simulink model "IEEE14_case"  (R2024b)
settings: Solver=FixedStepAuto  StartTime=0  StopTime=2  FixedStep=1e-7  RelTol=1e-3
values from neighbouring files (symbols this model uses):
  GFL_15_Bva = 0.009    [IEEE14_parameters.m]
  GFL_15_C_bus_pu = 7.179419    [IEEE14_parameters.m]
  GFL_15_f0 = 60    [IEEE14_parameters.m]
  GFL_15_I_id = 691.26967    [IEEE14_parameters.m]
  GFL_15_I_iq = 691.26967    [IEEE14_parameters.m]
  GFL_15_I_od = 45.2207    [IEEE14_parameters.m]
  GFL_15_I_oq = 45.2207    [IEEE14_parameters.m]
  GFL_15_I_pll = 0.78    [IEEE14_parameters.m]
  GFL_15_Kdi = 0.09    [IEEE14_parameters.m]
  GFL_15_Kdo = 0.9    [IEEE14_parameters.m]
  GFL_15_Kqi = 0.09    [IEEE14_parameters.m]
  GFL_15_Kqo = 0.9    [IEEE14_parameters.m]
  GFL_15_Lg_pu = 0.631447    [IEEE14_parameters.m]
  GFL_15_mode = 1    [IEEE14_parameters.m]
  GFL_15_P_id = 3.7166    [IEEE14_parameters.m]
  GFL_15_P_iq = 3.7166    [IEEE14_parameters.m]
  GFL_15_P_od = 0.4798    [IEEE14_parameters.m]
  GFL_15_P_oq = 0.4798    [IEEE14_parameters.m]
  GFL_15_P_pll = 290.42    [IEEE14_parameters.m]
  GFL_15_Qe_ref = 0.2    [IEEE14_parameters.m]
  GFL_15_Rg_pu = 0.024016    [IEEE14_parameters.m]
  GFL_15_Sbase = 1.000000e+4    (= 10000)    [IEEE14_parameters.m]
  GFL_15_Tdi = 0.01    [IEEE14_parameters.m]
  GFL_15_Tdo = 0.2    [IEEE14_parameters.m]
  GFL_15_Tqi = 0.01    [IEEE14_parameters.m]
  GFL_15_Tqo = 0.2    [IEEE14_parameters.m]
  GFL_15_Vbase = 380    [IEEE14_parameters.m]
  GFL_15_Vdc_ref = 1.011475    [IEEE14_parameters.m]
  GFL_15_Vdcbase = 700    [IEEE14_parameters.m]
  GFL_15_vq_ref = 0    [IEEE14_parameters.m]
  GFL_16_Bva = 0.002    [IEEE14_parameters.m]
  GFL_16_C_bus_pu = 7.179419    [IEEE14_parameters.m]
  GFL_16_f0 = 60    [IEEE14_parameters.m]
  GFL_16_I_id = 691.26967    [IEEE14_parameters.m]
  GFL_16_I_iq = 691.26967    [IEEE14_parameters.m]
  GFL_16_I_od = 45.2207    [IEEE14_parameters.m]
  GFL_16_I_oq = 45.2207    [IEEE14_parameters.m]
  GFL_16_I_pll = 0.78    [IEEE14_parameters.m]
  GFL_16_Kdi = 0.05    [IEEE14_parameters.m]
  GFL_16_Kdo = 0.5    [IEEE14_parameters.m]
  GFL_16_Kqi = 0.05    [IEEE14_parameters.m]
  GFL_16_Kqo = 0.5    [IEEE14_parameters.m]
  GFL_16_Lg_pu = 0.631447    [IEEE14_parameters.m]
  GFL_16_mode = 1    [IEEE14_parameters.m]
  GFL_16_P_id = 3.7166    [IEEE14_parameters.m]
  GFL_16_P_iq = 3.7166    [IEEE14_parameters.m]
  GFL_16_P_od = 0.4798    [IEEE14_parameters.m]
  GFL_16_P_oq = 0.4798    [IEEE14_parameters.m]
  GFL_16_P_pll = 290.42    [IEEE14_parameters.m]
  GFL_16_Qe_ref = 0.2    [IEEE14_parameters.m]
  GFL_16_Rg_pu = 0.024016    [IEEE14_parameters.m]
  GFL_16_Sbase = 1.000000e+4    (= 10000)    [IEEE14_parameters.m]
  GFL_16_Tdi = 0.01    [IEEE14_parameters.m]
  GFL_16_Tdo = 0.2    [IEEE14_parameters.m]
  GFL_16_Tqi = 0.01    [IEEE14_parameters.m]
  GFL_16_Tqo = 0.2    [IEEE14_parameters.m]
  GFL_16_Vbase = 380    [IEEE14_parameters.m]
  GFL_16_Vdc_ref = 1.01144    [IEEE14_parameters.m]
  GFL_16_Vdcbase = 700    [IEEE14_parameters.m]
  GFL_16_vq_ref = 0    [IEEE14_parameters.m]
  GFL_17_Bva = 0.002    [IEEE14_parameters.m]
  GFL_17_C_bus_pu = 7.179419    [IEEE14_parameters.m]
  GFL_17_f0 = 60    [IEEE14_parameters.m]
  GFL_17_I_id = 691.26967    [IEEE14_parameters.m]
  GFL_17_I_iq = 691.26967    [IEEE14_parameters.m]
  GFL_17_I_od = 45.2207    [IEEE14_parameters.m]
  GFL_17_I_oq = 45.2207    [IEEE14_parameters.m]
  GFL_17_I_pll = 0.78    [IEEE14_parameters.m]
  GFL_17_Kdi = 0.05    [IEEE14_parameters.m]
  GFL_17_Kdo = 0.5    [IEEE14_parameters.m]
  GFL_17_Kqi = 0.05    [IEEE14_parameters.m]
  GFL_17_Kqo = 0.5    [IEEE14_parameters.m]
  GFL_17_Lg_pu = 0.631447    [IEEE14_parameters.m]
  GFL_17_mode = 1    [IEEE14_parameters.m]
  GFL_17_P_id = 3.7166    [IEEE14_parameters.m]
  GFL_17_P_iq = 3.7166    [IEEE14_parameters.m]
  GFL_17_P_od = 0.4798    [IEEE14_parameters.m]
  GFL_17_P_oq = 0.4798    [IEEE14_parameters.m]
  GFL_17_P_pll = 290.42    [IEEE14_parameters.m]
  GFL_17_Qe_ref = 0.2    [IEEE14_parameters.m]
  GFL_17_Rg_pu = 0.024016    [IEEE14_parameters.m]
  GFL_17_Sbase = 1.000000e+4    (= 10000)    [IEEE14_parameters.m]
  GFL_17_Tdi = 0.01    [IEEE14_parameters.m]
  GFL_17_Tdo = 0.2    [IEEE14_parameters.m]
  GFL_17_Tqi = 0.01    [IEEE14_parameters.m]
  GFL_17_Tqo = 0.2    [IEEE14_parameters.m]
  GFL_17_Vbase = 380    [IEEE14_parameters.m]
  GFL_17_Vdc_ref = 1.011632    [IEEE14_parameters.m]
  GFL_17_Vdcbase = 700    [IEEE14_parameters.m]
  GFL_17_vq_ref = 0    [IEEE14_parameters.m]
  GFL_18_Bva = 0.002    [IEEE14_parameters.m]
  GFL_18_C_bus_pu = 7.179419    [IEEE14_parameters.m]
  GFL_18_f0 = 60    [IEEE14_parameters.m]
  GFL_18_I_id = 691.26967    [IEEE14_parameters.m]
  GFL_18_I_iq = 691.26967    [IEEE14_parameters.m]
  GFL_18_I_od = 45.2207    [IEEE14_parameters.m]
  GFL_18_I_oq = 45.2207    [IEEE14_parameters.m]
  GFL_18_I_pll = 0.78    [IEEE14_parameters.m]
  GFL_18_Kdi = 0.05    [IEEE14_parameters.m]
  GFL_18_Kdo = 0.5    [IEEE14_parameters.m]
  GFL_18_Kqi = 0.05    [IEEE14_parameters.m]
  GFL_18_Kqo = 0.5    [IEEE14_parameters.m]
  GFL_18_Lg_pu = 0.631447    [IEEE14_parameters.m]
  GFL_18_mode = 1    [IEEE14_parameters.m]
  GFL_18_P_id = 3.7166    [IEEE14_parameters.m]
  GFL_18_P_iq = 3.7166    [IEEE14_parameters.m]
  GFL_18_P_od = 0.4798    [IEEE14_parameters.m]
  GFL_18_P_oq = 0.4798    [IEEE14_parameters.m]
  GFL_18_P_pll = 290.42    [IEEE14_parameters.m]
  GFL_18_Qe_ref = 0.2    [IEEE14_parameters.m]
  GFL_18_Rg_pu = 0.024016    [IEEE14_parameters.m]
  GFL_18_Sbase = 1.000000e+4    (= 10000)    [IEEE14_parameters.m]
  GFL_18_Tdi = 0.01    [IEEE14_parameters.m]
  GFL_18_Tdo = 0.2    [IEEE14_parameters.m]
  GFL_18_Tqi = 0.01    [IEEE14_parameters.m]
  GFL_18_Tqo = 0.2    [IEEE14_parameters.m]
  GFL_18_Vbase = 380    [IEEE14_parameters.m]
  GFL_18_Vdc_ref = 1.011572    [IEEE14_parameters.m]
  GFL_18_Vdcbase = 700    [IEEE14_parameters.m]
  GFL_18_vq_ref = 0    [IEEE14_parameters.m]
  ... (+180 more)
(part 19 of 25)

== system IEEE14_case/SG_D_2/i_q_SG_D_2_block ==
  note: i_q_SG_D_2 in case14gfl
      | $-\frac{\sin\left(\theta _{\mathrm{SG},D,2}\right)\,\left(\psi _{q,\mathrm{SG},D,2}+\frac{\psi _{\mathrm{gq},\mathrm{SG},D,2}\,\left(x_{l}-x_{\mathrm{qdd}}\right)}{x_{l}-x_{\mathrm{qd}}}+\frac{\psi _{\mathrm{kq},\mathrm{SG},D,2}\,\left(x_{\mathrm{qd}}-x_{\mathrm{qdd}}\right)}{x_{l}-x_{\mathrm{qd}}}\right)}{x_{\mathrm{qdd}}}-\frac{\cos\left(\theta _{\mathrm{SG},D,2}\right)\,\left(\frac{\psi _{\mathrm{1d},\mathrm{SG},D,2}\,\left(x_{\mathrm{dd}}-x_{\mathrm{ddd}}\right)}{x_{\mathrm{dd}}-x_{l}}-\psi _{d,\mathrm{SG},D,2}+\frac{\psi _{\mathrm{fd},\mathrm{SG},D,2}\,\left(x_{\mathrm{ddd}}-x_{l}\right)}{x_{\mathrm{dd}}-x_{l}}\right)}{x_{\mathrm{ddd}}}$
      | Automatically generated on 2025-10-09 21:31:35 .
  State_psi_gq_SG_D_2_7930d : Inport
  State_psi_kq_SG_D_2_485e8 : Inport  Port=2
  State_psi_q_SG_D_2_38e4d : Inport  Port=3
  State_theta_SG_D_2_4758d : Inport  Port=4
  State_psi_1d_SG_D_2_da86a : Inport  Port=5
  State_psi_d_SG_D_2_afab4 : Inport  Port=6
  State_psi_fd_SG_D_2_93752 : Inport  Port=7
  State_theta_SG_D_2_47d8a : Inport  Port=8
  Add_21d4d : Sum
  Add_4c702 : Sum
  Add_61a1f : Sum
  Add_93cfc : Sum
  Add_a0bc2 : Sum
  Add_c78ca : Sum
  Constant_-1_29293 : Constant  Value=-1
  Constant_-1_bff13 : Constant  Value=-1
  Constant_-1_c93ee : Constant  Value=-1
  Constant_-1_d10ec : Constant  Value=-1
  Constant_-1_ff051 : Constant  Value=-1
  Constant_x_dd_48c29 : Constant  Value=x_dd
  Constant_x_dd_90d16 : Constant  Value=x_dd
  Constant_x_dd_c21b4 : Constant  Value=x_dd
  Constant_x_ddd_17e72 : Constant  Value=x_ddd
  Constant_x_ddd_23313 : Constant  Value=x_ddd
  Constant_x_ddd_882f4 : Constant  Value=x_ddd
  Constant_x_l_5f0ad : Constant  Value=x_l
  Constant_x_l_7718c : Constant  Value=x_l
  Constant_x_l_848fb : Constant  Value=x_l
  Constant_x_l_bf522 : Constant  Value=x_l
  Constant_x_l_da4ea : Constant  Value=x_l
  Constant_x_l_fd2ea : Constant  Value=x_l
  Constant_x_qd_1c516 : Constant  Value=x_qd
  Constant_x_qd_6b8e4 : Constant  Value=x_qd
  Constant_x_qd_ab2f4 : Constant  Value=x_qd
  Constant_x_qdd_2efaf : Constant  Value=x_qdd
  Constant_x_qdd_4f259 : Constant  Value=x_qdd
  Constant_x_qdd_8f0d3 : Constant  Value=x_qdd
  Divide_0d98a : Product  Inputs=*/
  Divide_6686b : Product  Inputs=*/
  Divide_800fc : Product  Inputs=*/
  Divide_af4a4 : Product  Inputs=*/
  Divide_c2bfd : Product  Inputs=*/
  Divide_c7e7f : Product  Inputs=*/
  MathFunc_cos_01a92 : Trigonometry  Operator=cos
  MathFunc_sin_e2c9e : Trigonometry
  Product_154d0 : Product
  Product_2c8d6 : Product
  Product_3fca9 : Product
  Product_44d62 : Product
  Product_5833b : Product
  Product_5d3bb : Product
  Product_68f6e : Product
  Product_97475 : Product
  Product_a96ba : Product
  Product_d2e3e : Product
  Product_fefb9 : Product
  Subtract_1a000 : Sum  Inputs=+-
  Subtract_2a5b7 : Sum  Inputs=+-
  Subtract_52633 : Sum  Inputs=+-
  Subtract_7c24d : Sum  Inputs=+-
  Subtract_cfdc8 : Sum  Inputs=+-
  Subtract_ecb99 : Sum  Inputs=+-
  Subtract_f70f0 : Sum  Inputs=+-
  Blockout_i_q_SG_D_2_d03bb : Outport
  wires:
  MathFunc_sin_e2c9e/1 -> Product_5d3bb/2
  Product_fefb9/1 -> Product_5d3bb/1
  Constant_-1_d10ec/1 -> Product_68f6e/1
  Constant_-1_c93ee/1 -> Product_2c8d6/1
  Constant_x_l_bf522/1 -> Product_68f6e/2
  Product_68f6e/1 -> Add_21d4d/1
  Subtract_f70f0/1 -> Product_d2e3e/2
  Constant_x_qdd_4f259/1 -> Subtract_ecb99/2
  Constant_x_qdd_2efaf/1 -> Add_21d4d/2
  Add_93cfc/1 -> Product_fefb9/2
  Constant_x_l_848fb/1 -> Product_2c8d6/2
  Constant_x_qd_ab2f4/1 -> Subtract_ecb99/1
  Constant_-1_ff051/1 -> Product_154d0/1
  Constant_x_l_da4ea/1 -> Product_154d0/2
  State_psi_1d_SG_D_2_da86a/1 -> Product_3fca9/2
  State_psi_gq_SG_D_2_7930d/1 -> Product_a96ba/1
  Add_21d4d/1 -> Product_a96ba/2
  Product_2c8d6/1 -> Add_c78ca/1
  Divide_c2bfd/1 -> Add_a0bc2/1
  Constant_x_qd_6b8e4/1 -> Add_c78ca/2
  State_psi_kq_SG_D_2_485e8/1 -> Product_97475/1
  Add_4c702/1 -> Subtract_2a5b7/1
  Constant_x_ddd_23313/1 -> Subtract_f70f0/2
  Subtract_ecb99/1 -> Product_97475/2
  Product_154d0/1 -> Add_61a1f/1
  Constant_x_qd_1c516/1 -> Add_61a1f/2
  Constant_-1_bff13/1 -> Product_3fca9/1
  Constant_x_l_7718c/1 -> Subtract_cfdc8/2
  Constant_x_dd_c21b4/1 -> Subtract_f70f0/1
  Product_a96ba/1 -> Divide_6686b/1
  Divide_c7e7f/1 -> Subtract_2a5b7/2
  Add_c78ca/1 -> Divide_6686b/2
  Product_44d62/1 -> Divide_0d98a/1
  Product_97475/1 -> Divide_af4a4/1
  Constant_-1_29293/1 -> Product_fefb9/1
  Product_3fca9/1 -> Product_d2e3e/1
  Add_61a1f/1 -> Divide_af4a4/2
  Constant_x_dd_48c29/1 -> Subtract_52633/1
  Subtract_2a5b7/1 -> Product_44d62/1
  Subtract_1a000/1 -> Product_5833b/2
  Constant_x_l_fd2ea/1 -> Subtract_52633/2
  Constant_x_ddd_882f4/1 -> Subtract_1a000/1
  Constant_x_l_5f0ad/1 -> Subtract_1a000/2
  Divide_6686b/1 -> Subtract_7c24d/1
  Divide_0d98a/1 -> Add_a0bc2/2
  Product_5833b/1 -> Divide_c7e7f/1
  Divide_af4a4/1 -> Subtract_7c24d/2
  Subtract_cfdc8/1 -> Divide_c7e7f/2
  Product_d2e3e/1 -> Divide_800fc/1
  Subtract_52633/1 -> Divide_800fc/2
  Constant_x_qdd_8f0d3/1 -> Divide_c2bfd/2
  State_psi_fd_SG_D_2_93752/1 -> Product_5833b/1
  Constant_x_dd_90d16/1 -> Subtract_cfdc8/1
  Subtract_7c24d/1 -> Add_93cfc/1
  State_psi_q_SG_D_2_38e4d/1 -> Add_93cfc/2
  Constant_x_ddd_17e72/1 -> Divide_0d98a/2
  Divide_800fc/1 -> Add_4c702/1
  State_psi_d_SG_D_2_afab4/1 -> Add_4c702/2
  State_theta_SG_D_2_4758d/1 -> MathFunc_sin_e2c9e/1
  State_theta_SG_D_2_47d8a/1 -> MathFunc_cos_01a92/1
  MathFunc_cos_01a92/1 -> Product_44d62/2
  Product_5d3bb/1 -> Divide_c2bfd/1
  Add_a0bc2/1 -> Blockout_i_q_SG_D_2_d03bb/1

== system IEEE14_case/SG_D_2/theta_SG_D_2_out_block ==
  note: theta_SG_D_2_out in case14gfl
      | $\theta _{\mathrm{SG},D,2}$
      | Automatically generated on 2025-10-09 21:31:39 .
  State_theta_SG_D_2_36941 : Inport
  Blockout_theta_SG_D_2_out_85337 : Outport
  wires:
  State_theta_SG_D_2_36941/1 -> Blockout_theta_SG_D_2_out_85337/1

== system IEEE14_case/SG_D_2/w_SG_D_2_out_block ==
  note: w_SG_D_2_out in case14gfl
      | $w_{\mathrm{SG},D,2}$
      | Automatically generated on 2025-10-09 21:31:39 .
  State_w_SG_D_2_35bfa : Inport
  Blockout_w_SG_D_2_out_7dd39 : Outport
  wires:
  State_w_SG_D_2_35bfa/1 -> Blockout_w_SG_D_2_out_7dd39/1

== system IEEE14_case/SG_D_3/T_e_SG_D_3_block ==
  note: T_e_SG_D_3 in case14gfl
      | $-\frac{\psi _{d,\mathrm{SG},D,3}\,\left(\psi _{q,\mathrm{SG},D,3}+\frac{\psi _{\mathrm{gq},\mathrm{SG},D,3}\,\left(x_{l}-x_{\mathrm{qdd}}\right)}{x_{l}-x_{\mathrm{qd}}}+\frac{\psi _{\mathrm{kq},\mathrm{SG},D,3}\,\left(x_{\mathrm{qd}}-x_{\mathrm{qdd}}\right)}{x_{l}-x_{\mathrm{qd}}}\right)}{x_{\mathrm{qdd}}}-\frac{\psi _{q,\mathrm{SG},D,3}\,\left(\frac{\psi _{\mathrm{1d},\mathrm{SG},D,3}\,\left(x_{\mathrm{dd}}-x_{\mathrm{ddd}}\right)}{x_{\mathrm{dd}}-x_{l}}-\psi _{d,\mathrm{SG},D,3}+\frac{\psi _{\mathrm{fd},\mathrm{SG},D,3}\,\left(x_{\mathrm{ddd}}-x_{l}\right)}{x_{\mathrm{dd}}-x_{l}}\right)}{x_{\mathrm{ddd}}}$
      | Automatically generated on 2025-10-09 21:32:38 .
  State_psi_d_SG_D_3_0fe66 : Inport
  State_psi_gq_SG_D_3_9f172 : Inport  Port=2
  State_psi_kq_SG_D_3_a8962 : Inport  Port=3
  State_psi_q_SG_D_3_e8f69 : Inport  Port=4
  State_psi_q_SG_D_3_454dd : Inport  Port=5
  State_psi_1d_SG_D_3_7e2e9 : Inport  Port=6
  State_psi_d_SG_D_3_9c5b0 : Inport  Port=7
  State_psi_fd_SG_D_3_2a972 : Inport  Port=8
  Add_09014 : Sum
  Add_394a0 : Sum
  Add_7224c : Sum
  Add_8082b : Sum
  Add_a05d9 : Sum
  Add_e10c3 : Sum
  Constant_-1_01911 : Constant  Value=-1
  Constant_-1_0cd0b : Constant  Value=-1
  Constant_-1_74786 : Constant  Value=-1
  Constant_-1_da5fd : Constant  Value=-1
  Constant_-1_fc2cc : Constant  Value=-1
  Constant_x_dd_4daa3 : Constant  Value=x_dd
  Constant_x_dd_55e1e : Constant  Value=x_dd
  Constant_x_dd_ac593 : Constant  Value=x_dd
  Constant_x_ddd_0ea54 : Constant  Value=x_ddd
  Constant_x_ddd_9de12 : Constant  Value=x_ddd
  Constant_x_ddd_eb100 : Constant  Value=x_ddd
  Constant_x_l_4ae37 : Constant  Value=x_l
  Constant_x_l_a1325 : Constant  Value=x_l
  Constant_x_l_bb800 : Constant  Value=x_l
  Constant_x_l_d6542 : Constant  Value=x_l
  Constant_x_l_e0126 : Constant  Value=x_l
  Constant_x_l_f24ed : Constant  Value=x_l
  Constant_x_qd_0f6ca : Constant  Value=x_qd
  Constant_x_qd_2c127 : Constant  Value=x_qd
  Constant_x_qd_2db5a : Constant  Value=x_qd
  Constant_x_qdd_4c195 : Constant  Value=x_qdd
  Constant_x_qdd_59a6b : Constant  Value=x_qdd
  Constant_x_qdd_ba1b8 : Constant  Value=x_qdd
  Divide_0efd0 : Product  Inputs=*/
  Divide_33e58 : Product  Inputs=*/
  Divide_4faf8 : Product  Inputs=*/
  Divide_82dd5 : Product  Inputs=*/
  Divide_894ca : Product  Inputs=*/
  Divide_d7dd3 : Product  Inputs=*/
  Product_0a5c8 : Product
  Product_1c6a3 : Product
  Product_35499 : Product
  Product_52b62 : Product
  Product_541b9 : Product
  Product_9c6e2 : Product
  Product_b46ac : Product
  Product_bff99 : Product
  Product_cc772 : Product
  Product_db715 : Product
  Product_efb59 : Product
  Subtract_0ea64 : Sum  Inputs=+-
  Subtract_21c6f : Sum  Inputs=+-
  Subtract_426c8 : Sum  Inputs=+-
  Subtract_6d66b : Sum  Inputs=+-
  Subtract_71cf7 : Sum  Inputs=+-
  Subtract_85126 : Sum  Inputs=+-
  Subtract_b8cec : Sum  Inputs=+-
  Blockout_T_e_SG_D_3_eef6a : Outport
  wires:
  State_psi_q_SG_D_3_e8f69/1 -> Add_e10c3/2
  Constant_-1_fc2cc/1 -> Product_cc772/1
  Subtract_21c6f/1 -> Product_bff99/2
  State_psi_1d_SG_D_3_7e2e9/1 -> Product_b46ac/2
  Constant_-1_0cd0b/1 -> Product_52b62/1
  Constant_x_l_4ae37/1 -> Product_52b62/2
  Add_7224c/1 -> Subtract_21c6f/1
  State_psi_d_SG_D_3_9c5b0/1 -> Add_7224c/2
  Product_52b62/1 -> Add_394a0/1
  Constant_x_qdd_ba1b8/1 -> Subtract_71cf7/2
  Add_e10c3/1 -> Product_1c6a3/2
  Constant_x_qdd_59a6b/1 -> Add_394a0/2
  State_psi_q_SG_D_3_454dd/1 -> Product_bff99/1
  Constant_x_l_e0126/1 -> Product_cc772/2
  Subtract_0ea64/1 -> Divide_82dd5/2
  Constant_x_l_f24ed/1 -> Subtract_85126/2
  Constant_x_qd_0f6ca/1 -> Subtract_71cf7/1
  Constant_-1_da5fd/1 -> Product_efb59/1
  Subtract_426c8/1 -> Divide_33e58/2
  Constant_x_l_a1325/1 -> Product_efb59/2
  Product_541b9/1 -> Divide_33e58/1
  Constant_-1_01911/1 -> Product_b46ac/1
  Product_b46ac/1 -> Product_541b9/1
  Constant_x_dd_55e1e/1 -> Subtract_b8cec/1
  Constant_x_ddd_eb100/1 -> Subtract_b8cec/2
  Add_09014/1 -> Blockout_T_e_SG_D_3_eef6a/1
  State_psi_gq_SG_D_3_9f172/1 -> Product_0a5c8/1
  Product_bff99/1 -> Divide_0efd0/1
  Add_394a0/1 -> Product_0a5c8/2
  State_psi_fd_SG_D_3_2a972/1 -> Product_9c6e2/1
  Product_cc772/1 -> Add_a05d9/1
  Constant_x_qd_2c127/1 -> Add_a05d9/2
  Constant_x_dd_4daa3/1 -> Subtract_426c8/1
  State_psi_kq_SG_D_3_a8962/1 -> Product_db715/1
  Constant_x_dd_ac593/1 -> Subtract_0ea64/1
  Subtract_71cf7/1 -> Product_db715/2
  Product_1c6a3/1 -> Divide_d7dd3/1
  Product_efb59/1 -> Add_8082b/1
  Add_a05d9/1 -> Divide_894ca/2
  Constant_x_qd_2db5a/1 -> Add_8082b/2
  Subtract_b8cec/1 -> Product_541b9/2
  Constant_x_l_bb800/1 -> Subtract_426c8/2
  Constant_x_ddd_9de12/1 -> Subtract_85126/1
  Product_0a5c8/1 -> Divide_894ca/1
  Product_db715/1 -> Divide_4faf8/1
  Add_8082b/1 -> Divide_4faf8/2
  Constant_x_ddd_0ea54/1 -> Divide_0efd0/2
  Subtract_85126/1 -> Product_9c6e2/2
  Divide_894ca/1 -> Subtract_6d66b/1
  Constant_x_l_d6542/1 -> Subtract_0ea64/2
  Divide_4faf8/1 -> Subtract_6d66b/2
  Divide_33e58/1 -> Add_7224c/1
  Product_9c6e2/1 -> Divide_82dd5/1
  Constant_-1_74786/1 -> Product_35499/1
  State_psi_d_SG_D_3_0fe66/1 -> Product_35499/2
  Subtract_6d66b/1 -> Add_e10c3/1
  Divide_82dd5/1 -> Subtract_21c6f/2
  Product_35499/1 -> Product_1c6a3/1
  Constant_x_qdd_4c195/1 -> Divide_d7dd3/2
  Divide_d7dd3/1 -> Add_09014/1
  Divide_0efd0/1 -> Add_09014/2

== system IEEE14_case/SG_D_3/d_E_fd_SG_D_3_block ==
  note: d_E_fd_SG_D_3 in case14gfl
      | $\frac{V_{f,\mathrm{SG},D,3}-E_{\mathrm{fd},\mathrm{SG},D,3}\,K_{E}}{T_{E}}$
      | Automatically generated on 2025-10-09 21:32:24 .
  State_E_fd_SG_D_3_7ac9b : Inport
  State_V_f_SG_D_3_89c49 : Inport  Port=2
  Add_8d57b : Sum
  Constant_-1_53129 : Constant  Value=-1
  Constant_K_E_6c208 : Constant  Value=K_E
  Constant_T_E_f95db : Constant  Value=T_E
  Divide_bae81 : Product  Inputs=*/
  Product_40f1c : Product
  Product_529fa : Product
  Blockout_d_E_fd_SG_D_3_cf470 : Outport
  wires:
  State_V_f_SG_D_3_89c49/1 -> Add_8d57b/2
  Constant_-1_53129/1 -> Product_529fa/1
  State_E_fd_SG_D_3_7ac9b/1 -> Product_529fa/2
  Constant_T_E_f95db/1 -> Divide_bae81/2
  Product_529fa/1 -> Product_40f1c/1
  Product_40f1c/1 -> Add_8d57b/1
  Constant_K_E_6c208/1 -> Product_40f1c/2
  Divide_bae81/1 -> Blockout_d_E_fd_SG_D_3_cf470/1
  Add_8d57b/1 -> Divide_bae81/1

== system IEEE14_case/SG_D_3/d_Px_1_SG_D_3_block ==
  note: d_Px_1_SG_D_3 in case14gfl
      | $\frac{w_{\mathrm{SG},D,3}-2\,\pi \,f_{0}}{T_{w}}-\frac{\mathrm{Px}_{1,\mathrm{SG},D,3}}{T_{w}}$
      | Automatically generated on 2025-10-09 21:32:25 .
  State_Px_1_SG_D_3_31f88 : Inport
  State_w_SG_D_3_8df22 : Inport  Port=2
  Add_1cf09 : Sum
  Add_50941 : Sum
  Constant_-1_b31d5 : Constant  Value=-1
  Constant_-2.0_37952 : Constant  Value=-2.0
  Constant_T_w_a3fb0 : Constant  Value=T_w
  Constant_T_w_e3553 : Constant  Value=T_w
  Constant_f0_02273 : Constant  Value=f0
  Constant_pi_1df47 : Constant  Value=pi
  Divide_46959 : Product  Inputs=*/
  Divide_ce75d : Product  Inputs=*/
  Product_3990a : Product
  Product_6a5b3 : Product
  Product_90ff5 : Product
  Blockout_d_Px_1_SG_D_3_2db33 : Outport
  wires:
  Constant_f0_02273/1 -> Product_90ff5/2
  Constant_-1_b31d5/1 -> Product_6a5b3/1
  Constant_-2.0_37952/1 -> Product_3990a/1
  Constant_pi_1df47/1 -> Product_3990a/2
  Product_3990a/1 -> Product_90ff5/1
  State_w_SG_D_3_8df22/1 -> Add_1cf09/2
  Divide_ce75d/1 -> Add_50941/1
  State_Px_1_SG_D_3_31f88/1 -> Product_6a5b3/2
  Product_90ff5/1 -> Add_1cf09/1
  Product_6a5b3/1 -> Divide_ce75d/1
  Constant_T_w_a3fb0/1 -> Divide_ce75d/2
  Add_1cf09/1 -> Divide_46959/1
  Constant_T_w_e3553/1 -> Divide_46959/2
  Divide_46959/1 -> Add_50941/2
  Add_50941/1 -> Blockout_d_Px_1_SG_D_3_2db33/1

== system IEEE14_case/SG_D_3/d_Px_2_SG_D_3_block ==
  note: d_Px_2_SG_D_3 in case14gfl
      | $\frac{\mathrm{Px}_{1,\mathrm{SG},D,3}-T_{2}\,\left(\frac{\mathrm{Px}_{1,\mathrm{SG},D,3}}{T_{w}}-\frac{w_{\mathrm{SG},D,3}-2\,\pi \,f_{0}}{T_{w}}\right)}{T_{1}}-\frac{\mathrm{Px}_{2,\mathrm{SG},D,3}}{T_{1}}$
      | Automatically generated on 2025-10-09 21:32:26 .
  State_Px_2_SG_D_3_c0631 : Inport
  State_Px_1_SG_D_3_9548d : Inport  Port=2
  State_Px_1_SG_D_3_76f6d : Inport  Port=3
  State_w_SG_D_3_c1cd3 : Inport  Port=4
  Add_7696a : Sum
  Add_9c22b : Sum
  Add_e8c5d : Sum
  Add_f607d : Sum
  Constant_-1_3a112 : Constant  Value=-1
  Constant_-1_3bd98 : Constant  Value=-1
  Constant_-2.0_5772f : Constant  Value=-2.0
  Constant_T_1_3069d : Constant  Value=T_1
  Constant_T_1_ea066 : Constant  Value=T_1
  Constant_T_2_fc22f : Constant  Value=T_2
  Constant_T_w_1275a : Constant  Value=T_w
  Constant_T_w_d0e0d : Constant  Value=T_w
  Constant_f0_23775 : Constant  Value=f0
  Constant_pi_7d668 : Constant  Value=pi
  Divide_9514e : Product  Inputs=*/
  Divide_aab42 : Product  Inputs=*/
  Divide_cf3b8 : Product  Inputs=*/
  Divide_d6d97 : Product  Inputs=*/
  Product_16328 : Product
  Product_317d2 : Product
  Product_8ed5f : Product
  Product_bf14c : Product
  Product_f4b95 : Product
  Blockout_d_Px_2_SG_D_3_ebaee : Outport
  wires:
  State_Px_1_SG_D_3_76f6d/1 -> Product_f4b95/2
  Constant_-2.0_5772f/1 -> Product_16328/1
  Constant_f0_23775/1 -> Product_8ed5f/2
  Constant_pi_7d668/1 -> Product_16328/2
  Product_16328/1 -> Product_8ed5f/1
  State_w_SG_D_3_c1cd3/1 -> Add_9c22b/2
  Constant_-1_3bd98/1 -> Product_f4b95/1
  Product_8ed5f/1 -> Add_9c22b/1
  Product_f4b95/1 -> Divide_aab42/1
  Constant_T_w_1275a/1 -> Divide_aab42/2
  Add_9c22b/1 -> Divide_cf3b8/1
  Constant_T_w_d0e0d/1 -> Divide_cf3b8/2
  Divide_aab42/1 -> Add_e8c5d/1
  Divide_cf3b8/1 -> Add_e8c5d/2
  Constant_T_2_fc22f/1 -> Product_bf14c/1
  Add_e8c5d/1 -> Product_bf14c/2
  Constant_-1_3a112/1 -> Product_317d2/1
  Product_bf14c/1 -> Add_f607d/2
  State_Px_2_SG_D_3_c0631/1 -> Product_317d2/2
  State_Px_1_SG_D_3_9548d/1 -> Add_f607d/1
  Product_317d2/1 -> Divide_d6d97/1
  Add_7696a/1 -> Blockout_d_Px_2_SG_D_3_ebaee/1
  Constant_T_1_3069d/1 -> Divide_d6d97/2
  Add_f607d/1 -> Divide_9514e/1
  Constant_T_1_ea066/1 -> Divide_9514e/2
  Divide_d6d97/1 -> Add_7696a/1
  Divide_9514e/1 -> Add_7696a/2

== system IEEE14_case/SG_D_3/d_Px_3_SG_D_3_block ==
  note: d_Px_3_SG_D_3 in case14gfl
      | $\frac{\mathrm{Px}_{2,\mathrm{SG},D,3}+T_{4}\,\left(\frac{\mathrm{Px}_{1,\mathrm{SG},D,3}-T_{2}\,\left(\frac{\mathrm{Px}_{1,\mathrm{SG},D,3}}{T_{w}}-\frac{w_{\mathrm{SG},D,3}-2\,\pi \,f_{0}}{T_{w}}\right)}{T_{1}}-\frac{\mathrm{Px}_{2,\mathrm{SG},D,3}}{T_{1}}\right)}{T_{3}}-\frac{\mathrm{Px}_{3,\mathrm{SG},D,3}}{T_{3}}$
      | Automatically generated on 2025-10-09 21:32:29 .
  State_Px_3_SG_D_3_af481 : Inport
  State_Px_2_SG_D_3_c14d3 : Inport  Port=2
  State_Px_2_SG_D_3_bc145 : Inport  Port=3
  State_Px_1_SG_D_3_ffa71 : Inport  Port=4
  State_Px_1_SG_D_3_1185a : Inport  Port=5
  State_w_SG_D_3_40967 : Inport  Port=6
  Add_3a825 : Sum
  Add_4cb3b : Sum
  Add_811ac : Sum
  Add_8f6ad : Sum
  Add_d0407 : Sum
  Add_f2b18 : Sum
  Constant_-1_66813 : Constant  Value=-1
  Constant_-1_73ddc : Constant  Value=-1
  Constant_-1_c9e73 : Constant  Value=-1
  Constant_-2.0_cbd12 : Constant  Value=-2.0
  Constant_T_1_a322d : Constant  Value=T_1
  Constant_T_1_e31fb : Constant  Value=T_1
  Constant_T_2_c55df : Constant  Value=T_2
  Constant_T_3_afa77 : Constant  Value=T_3
  Constant_T_3_bd696 : Constant  Value=T_3
  Constant_T_4_ca1bc : Constant  Value=T_4
  Constant_T_w_2ac25 : Constant  Value=T_w
  Constant_T_w_4cb13 : Constant  Value=T_w
  Constant_f0_05acc : Constant  Value=f0
  Constant_pi_c0a43 : Constant  Value=pi
  Divide_2b38e : Product  Inputs=*/
  Divide_5aa4c : Product  Inputs=*/
  Divide_7e51e : Product  Inputs=*/
  Divide_b1903 : Product  Inputs=*/
  Divide_d9cb5 : Product  Inputs=*/
  Divide_e3570 : Product  Inputs=*/
  Product_1da24 : Product
  Product_8fcea : Product
  Product_9b954 : Product
  Product_bc2ec : Product
  Product_d5ac3 : Product
  Product_e3691 : Product
  Product_ece68 : Product
  Blockout_d_Px_3_SG_D_3_533e8 : Outport
  wires:
  State_Px_1_SG_D_3_1185a/1 -> Product_d5ac3/2
  Constant_f0_05acc/1 -> Product_ece68/2
  Constant_-2.0_cbd12/1 -> Product_8fcea/1
  Add_811ac/1 -> Divide_e3570/1
  Constant_pi_c0a43/1 -> Product_8fcea/2
  Product_8fcea/1 -> Product_ece68/1
  State_w_SG_D_3_40967/1 -> Add_8f6ad/2
  Constant_T_w_4cb13/1 -> Divide_7e51e/2
  Constant_-1_66813/1 -> Product_d5ac3/1
  Product_ece68/1 -> Add_8f6ad/1
  Product_d5ac3/1 -> Divide_7e51e/1
  Add_8f6ad/1 -> Divide_5aa4c/1
  Product_9b954/1 -> Divide_b1903/1
  Constant_T_w_2ac25/1 -> Divide_5aa4c/2
  Divide_7e51e/1 -> Add_d0407/1
  Divide_5aa4c/1 -> Add_d0407/2
  Constant_T_2_c55df/1 -> Product_e3691/1
  Add_d0407/1 -> Product_e3691/2
  Constant_-1_73ddc/1 -> Product_9b954/1
  State_Px_2_SG_D_3_bc145/1 -> Product_9b954/2
  State_Px_1_SG_D_3_ffa71/1 -> Add_811ac/1
  Constant_T_3_afa77/1 -> Divide_2b38e/2
  Product_e3691/1 -> Add_811ac/2
  Constant_T_1_a322d/1 -> Divide_b1903/2
  Add_3a825/1 -> Product_bc2ec/2
  Constant_T_1_e31fb/1 -> Divide_e3570/2
  Divide_d9cb5/1 -> Add_4cb3b/2
  Divide_b1903/1 -> Add_3a825/1
  Divide_e3570/1 -> Add_3a825/2
  Constant_T_4_ca1bc/1 -> Product_bc2ec/1
  Constant_-1_c9e73/1 -> Product_1da24/1
  State_Px_3_SG_D_3_af481/1 -> Product_1da24/2
  State_Px_2_SG_D_3_c14d3/1 -> Add_f2b18/1
  Product_bc2ec/1 -> Add_f2b18/2
  Product_1da24/1 -> Divide_2b38e/1
  Add_f2b18/1 -> Divide_d9cb5/1
  Constant_T_3_bd696/1 -> Divide_d9cb5/2
  Divide_2b38e/1 -> Add_4cb3b/1
  Add_4cb3b/1 -> Blockout_d_Px_3_SG_D_3_533e8/1

== system IEEE14_case/SG_D_3/d_R_f_SG_D_3_block ==
  note: d_R_f_SG_D_3 in case14gfl
      | $-\frac{R_{f,\mathrm{SG},D,3}-\frac{E_{\mathrm{fd},\mathrm{SG},D,3}\,K_{F}}{T_{F}}}{T_{F}}$
      | Automatically generated on 2025-10-09 21:32:23 .
  State_E_fd_SG_D_3_4b09f : Inport
  State_R_f_SG_D_3_eb135 : Inport  Port=2
  Constant_K_F_dd9b1 : Constant  Value=K_F
  Constant_T_F_11d51 : Constant  Value=T_F
  Constant_T_F_30861 : Constant  Value=T_F
  Divide_63da4 : Product  Inputs=*/
  Divide_ea8c5 : Product  Inputs=*/
  Product_1bbb6 : Product
  Subtract_6cec3 : Sum  Inputs=+-
  Blockout_d_R_f_SG_D_3_2588d : Outport
  wires:
  State_E_fd_SG_D_3_4b09f/1 -> Product_1bbb6/1
  Constant_T_F_30861/1 -> Divide_ea8c5/2
  Constant_K_F_dd9b1/1 -> Product_1bbb6/2
  Product_1bbb6/1 -> Divide_ea8c5/1
  Divide_ea8c5/1 -> Subtract_6cec3/1
  State_R_f_SG_D_3_eb135/1 -> Subtract_6cec3/2
  Subtract_6cec3/1 -> Divide_63da4/1
  Constant_T_F_11d51/1 -> Divide_63da4/2
  Divide_63da4/1 -> Blockout_d_R_f_SG_D_3_2588d/1

== system IEEE14_case/SG_D_3/d_T_m_SG_D_3_block ==
  note: d_T_m_SG_D_3 in case14gfl
      | $-\frac{T_{m,\mathrm{SG},D,3}-T_{0}+\frac{\mathrm{SpeedPara}\,\left(w_{\mathrm{SG},D,3}-w_{\mathrm{ref}}\right)}{2\,f_{0}\,\pi }}{T_{\mathrm{speed}}}$
      | Automatically generated on 2025-10-09 21:32:15 .
  State_w_SG_D_3_dca15 : Inport
  State_T_m_SG_D_3_13cc0 : Inport  Port=2
  Add_2e122 : Sum
  Add_a582f : Sum
  Constant_-1_1c454 : Constant  Value=-1
  Constant_2.0_125cb : Constant  Value=2.0
  Constant_SpeedPara_0c028 : Constant  Value=SpeedPara
  Constant_T_0_97111 : Constant  Value=T_0
  Constant_T_speed_fee19 : Constant  Value=T_speed
  Constant_f0_6dc78 : Constant  Value=f0
  Constant_pi_023ce : Constant  Value=pi
  Constant_w_ref_d9b59 : Constant  Value=w_ref
  Divide_32656 : Product  Inputs=*/
  Divide_a9f95 : Product  Inputs=*/
  Product_2ec29 : Product
  Product_a23e5 : Product
  Product_cf749 : Product
  Product_d540a : Product
  Subtract_cd11b : Sum  Inputs=+-
  Blockout_d_T_m_SG_D_3_ccb21 : Outport
  wires:
  Constant_SpeedPara_0c028/1 -> Product_cf749/1
  Constant_-1_1c454/1 -> Product_d540a/1
  Constant_w_ref_d9b59/1 -> Add_2e122/2
  State_w_SG_D_3_dca15/1 -> Product_d540a/2
  Constant_2.0_125cb/1 -> Product_a23e5/1
  Product_d540a/1 -> Add_2e122/1
  Constant_pi_023ce/1 -> Product_a23e5/2
  Add_2e122/1 -> Product_cf749/2
  Product_a23e5/1 -> Product_2ec29/1
  Constant_f0_6dc78/1 -> Product_2ec29/2
  Product_cf749/1 -> Divide_a9f95/1
  Product_2ec29/1 -> Divide_a9f95/2
  Divide_a9f95/1 -> Add_a582f/1
  Constant_T_0_97111/1 -> Add_a582f/2
  Add_a582f/1 -> Subtract_cd11b/1
  State_T_m_SG_D_3_13cc0/1 -> Subtract_cd11b/2
  Subtract_cd11b/1 -> Divide_32656/1
  Constant_T_speed_fee19/1 -> Divide_32656/2
  Divide_32656/1 -> Blockout_d_T_m_SG_D_3_ccb21/1

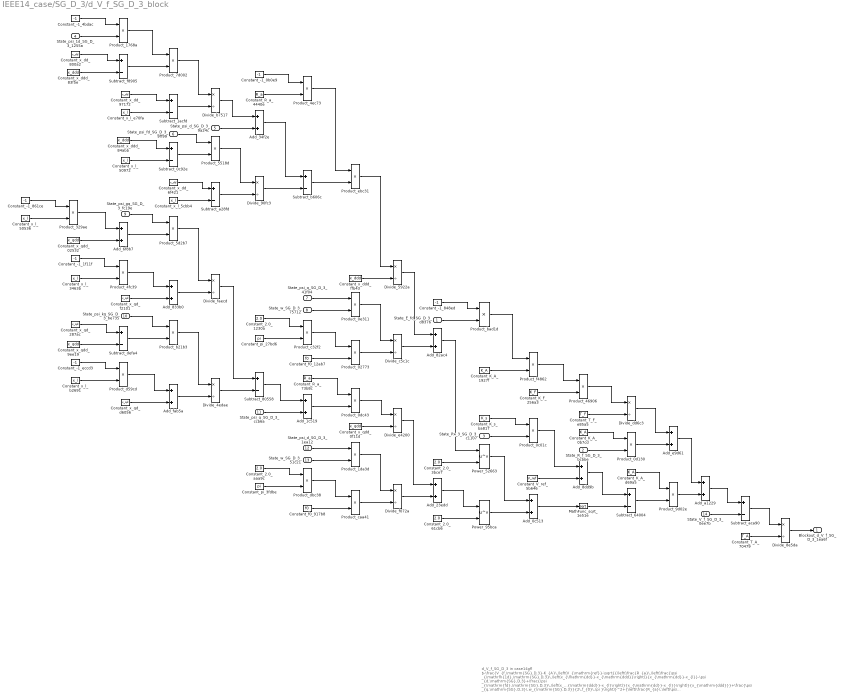
== system IEEE14_case/SG_D_3/d_V_f_SG_D_3_block ==
  note: d_V_f_SG_D_3 in case14gfl
      | $-\frac{V_{f,\mathrm{SG},D,3}-K_{A}\,\left(V_{\mathrm{ref}}-\sqrt{{\left(\frac{R_{a}\,\left(\frac{\psi _{\mathrm{1d},\mathrm{SG},D,3}\,\left(x_{\mathrm{dd}}-x_{\mathrm{ddd}}\right)}{x_{\mathrm{dd}}-x_{l}}-\psi _{d,\mathrm{SG},D,3}+\frac{\psi _{\mathrm{fd},\mathrm{SG},D,3}\,\left(x_{\mathrm{ddd}}-x_{l}\right)}{x_{\mathrm{dd}}-x_{l}}\right)}{x_{\mathrm{ddd}}}+\frac{\psi _{q,\mathrm{SG},D,3}\,w_{\mathrm{SG},D,3}}{2\,f_{0}\,\pi }\right)}^2+{\left(\frac{R_{a}\,\left(\psi _{q,\mathrm{SG},D,3}+\frac{\psi _{\mathrm{gq},\mathrm{SG},D,3}\,\left(x_{l}-x_{\mathrm{qdd}}\right)}{x_{l}-x_{\mathrm{qd}}}+\frac{\psi _{\mathrm{kq},\mathrm{SG},D,3}\,\left(x_{\mathrm{qd}}-x_{\mathrm{qdd}}\right)}{x_{l}-x_{\mathrm{qd}}}\right)}{x_{\mathrm{qdd}}}+\frac{\psi _{d,\mathrm{SG},D,3}\,w_{\mathrm{SG},D,3}}{2\,f_{0}\,\pi }\right)}^2}+K_{s}\,\mathrm{Px}_{3,\mathrm{SG},D,3}\right)-K_{A}\,R_{f,\mathrm{SG},D,3}+\frac{E_{\mathrm{fd},\mathrm{SG},D,3}\,K_{A}\,K_{F}}{T_{F}}}{T_{A}}$
      | Automatically generated on 2025-10-09 21:32:22 .
  State_E_fd_SG_D_3_d8376 : Inport
  State_R_f_SG_D_3_bcbbe : Inport  Port=2
  State_Px_3_SG_D_3_c1107 : Inport  Port=3
  State_psi_1d_SG_D_3_1255a : Inport  Port=4
  State_psi_d_SG_D_3_9a24c : Inport  Port=5
  State_psi_fd_SG_D_3_9ff99 : Inport  Port=6
  State_psi_q_SG_D_3_41f04 : Inport  Port=7
  State_w_SG_D_3_75712 : Inport  Port=8
  State_psi_gq_SG_D_3_fc19e : Inport  Port=9
  State_psi_kq_SG_D_3_be735 : Inport  Port=10
  State_psi_q_SG_D_3_ccb6a : Inport  Port=11
  State_psi_d_SG_D_3_1ea12 : Inport  Port=12
  State_w_SG_D_3_51c21 : Inport  Port=13
  State_V_f_SG_D_3_0ee7b : Inport  Port=14
  Add_0c513 : Sum
  Add_1c519 : Sum
  Add_23edd : Sum
  Add_34f2e : Sum
  Add_6f8b7 : Sum
  Add_82ac4 : Sum
  Add_833b0 : Sum
  Add_8dd9b : Sum
  Add_a1229 : Sum
  Add_e9d61 : Sum
  Add_fab5a : Sum
  Constant_-1_0b0e9 : Constant  Value=-1
  Constant_-1_1f11f : Constant  Value=-1
  Constant_-1_4bdac : Constant  Value=-1
  Constant_-1_848ed : Constant  Value=-1
  Constant_-1_861ce : Constant  Value=-1
  Constant_-1_eccd3 : Constant  Value=-1
  Constant_2.0_1230a : Constant  Value=2.0
  Constant_2.0_3bce7 : Constant  Value=2.0
  Constant_2.0_61cb6 : Constant  Value=2.0
  Constant_2.0_aaa9c : Constant  Value=2.0
  Constant_K_A_0b7cd : Constant  Value=K_A
  Constant_K_A_1927f : Constant  Value=K_A
  Constant_K_A_d69a5 : Constant  Value=K_A
  Constant_K_F_256a3 : Constant  Value=K_F
  Constant_K_s_ba817 : Constant  Value=K_s
  Constant_R_a_4440e : Constant  Value=R_a
  Constant_R_a_73b8c : Constant  Value=R_a
  Constant_T_A_70479 : Constant  Value=T_A
  Constant_T_F_e85a5 : Constant  Value=T_F
  Constant_V_ref_5b646 : Constant  Value=V_ref
  Constant_f0_12ab7 : Constant  Value=f0
  Constant_f0_917b8 : Constant  Value=f0
  Constant_pi_27bd6 : Constant  Value=pi
  Constant_pi_3fdbe : Constant  Value=pi
  Constant_x_dd_6f421 : Constant  Value=x_dd
  Constant_x_dd_800a2 : Constant  Value=x_dd
  Constant_x_dd_97172 : Constant  Value=x_dd
  Constant_x_ddd_83f5e : Constant  Value=x_ddd
  Constant_x_ddd_84abb : Constant  Value=x_ddd
  Constant_x_ddd_ffb43 : Constant  Value=x_ddd
  Constant_x_l_3463b : Constant  Value=x_l
  Constant_x_l_50536 : Constant  Value=x_l
  Constant_x_l_50972 : Constant  Value=x_l
  Constant_x_l_5cbb4 : Constant  Value=x_l
  Constant_x_l_b2691 : Constant  Value=x_l
  Constant_x_l_e70fa : Constant  Value=x_l
  Constant_x_qd_287ac : Constant  Value=x_qd
  Constant_x_qd_d6056 : Constant  Value=x_qd
  Constant_x_qd_f2101 : Constant  Value=x_qd
  Constant_x_qdd_02532 : Constant  Value=x_qdd
  Constant_x_qdd_0f11d : Constant  Value=x_qdd
  Constant_x_qdd_9ee19 : Constant  Value=x_qdd
  Divide_4edae : Product  Inputs=*/
  Divide_5922a : Product  Inputs=*/
  Divide_8e5da : Product  Inputs=*/
  Divide_90fc3 : Product  Inputs=*/
  Divide_b7517 : Product  Inputs=*/
  Divide_c5c1c : Product  Inputs=*/
  Divide_dd6c3 : Product  Inputs=*/
  Divide_e4200 : Product  Inputs=*/
  Divide_f072a : Product  Inputs=*/
  Divide_faecd : Product  Inputs=*/
  MathFunc_sqrt_1e51e : Sqrt
  Power_52663 : Math  Operator=pow
  Power_95bca : Math  Operator=pow
  Product_02773 : Product
  Product_0c01c : Product
  Product_0d130 : Product
  Product_0dc43 : Product
  Product_0e311 : Product
  Product_1768a : Product
  Product_1da3d : Product
  Product_329ae : Product
  Product_46906 : Product
  Product_4ec73 : Product
  Product_4fc39 : Product
  Product_5518d : Product
  Product_5d2b7 : Product
  Product_7d002 : Product
  Product_9d02e : Product
  Product_b21b3 : Product
  Product_bad1d : Product
  Product_c32f2 : Product
  Product_caa41 : Product
  Product_d59cd : Product
  Product_dbc38 : Product
  Product_ebc31 : Product
  Product_f4862 : Product
  Subtract_0c92e : Sum  Inputs=+-
  Subtract_1acfd : Sum  Inputs=+-
  Subtract_64004 : Sum  Inputs=+-
  Subtract_80558 : Sum  Inputs=+-
  Subtract_a28fd : Sum  Inputs=+-
  Subtract_aca90 : Sum  Inputs=+-
  Subtract_b606c : Sum  Inputs=+-
  Subtract_defa4 : Sum  Inputs=+-
  Subtract_f8905 : Sum  Inputs=+-
  Blockout_d_V_f_SG_D_3_1ea6f : Outport
  wires:
  Constant_K_A_0b7cd/1 -> Product_0d130/1
  Constant_-1_861ce/1 -> Product_329ae/1
  Subtract_0c92e/1 -> Product_5518d/2
  Constant_x_l_50536/1 -> Product_329ae/2
  Divide_f072a/1 -> Add_23edd/2
  Constant_-1_4bdac/1 -> Product_1768a/1
  State_psi_1d_SG_D_3_1255a/1 -> Product_1768a/2
  Constant_x_dd_800a2/1 -> Subtract_f8905/1
  Divide_90fc3/1 -> Subtract_b606c/2
  Product_329ae/1 -> Add_6f8b7/1
  Constant_x_qdd_02532/1 -> Add_6f8b7/2
  Constant_x_ddd_83f5e/1 -> Subtract_f8905/2
  Constant_2.0_61cb6/1 -> Power_95bca/2
  Constant_-1_1f11f/1 -> Product_4fc39/1
  Divide_faecd/1 -> Subtract_80558/1
  Subtract_1acfd/1 -> Divide_b7517/2
  Constant_x_l_3463b/1 -> Product_4fc39/2
  Constant_x_qd_287ac/1 -> Subtract_defa4/1
  State_w_SG_D_3_75712/1 -> Product_0e311/2
  Constant_x_qdd_9ee19/1 -> Subtract_defa4/2
  Constant_2.0_1230a/1 -> Product_c32f2/1
  Constant_-1_eccd3/1 -> Product_d59cd/1
  Constant_pi_27bd6/1 -> Product_c32f2/2
  Add_34f2e/1 -> Subtract_b606c/1
  Constant_x_l_b2691/1 -> Product_d59cd/2
  Product_1768a/1 -> Product_7d002/1
  Subtract_f8905/1 -> Product_7d002/2
  Constant_2.0_aaa9c/1 -> Product_dbc38/1
  Constant_x_dd_97172/1 -> Subtract_1acfd/1
  Constant_pi_3fdbe/1 -> Product_dbc38/2
  Constant_x_l_e70fa/1 -> Subtract_1acfd/2
  Constant_x_ddd_84abb/1 -> Subtract_0c92e/1
  Constant_x_l_50972/1 -> Subtract_0c92e/2
  State_psi_gq_SG_D_3_fc19e/1 -> Product_5d2b7/1
  Constant_x_l_5cbb4/1 -> Subtract_a28fd/2
  Add_6f8b7/1 -> Product_5d2b7/2
  Product_4fc39/1 -> Add_833b0/1
  Product_5d2b7/1 -> Divide_faecd/1
  Constant_x_qd_f2101/1 -> Add_833b0/2
  State_psi_kq_SG_D_3_be735/1 -> Product_b21b3/1
  State_psi_q_SG_D_3_41f04/1 -> Product_0e311/1
  Add_82ac4/1 -> Power_52663/1
  Subtract_defa4/1 -> Product_b21b3/2
  Constant_f0_12ab7/1 -> Product_02773/2
  Product_c32f2/1 -> Product_02773/1
  Constant_x_qd_d6056/1 -> Add_fab5a/2
  Product_d59cd/1 -> Add_fab5a/1
  Product_7d002/1 -> Divide_b7517/1
  State_psi_fd_SG_D_3_9ff99/1 -> Product_5518d/1
  Constant_x_dd_6f421/1 -> Subtract_a28fd/1
  Add_833b0/1 -> Divide_faecd/2
  Add_0c513/1 -> MathFunc_sqrt_1e51e/1
  Product_b21b3/1 -> Divide_4edae/1
  Add_fab5a/1 -> Divide_4edae/2
  Product_4ec73/1 -> Product_ebc31/1
  Divide_b7517/1 -> Add_34f2e/1
  Add_8dd9b/1 -> Subtract_64004/1
  State_psi_d_SG_D_3_9a24c/1 -> Add_34f2e/2
  Product_5518d/1 -> Divide_90fc3/1
  Subtract_a28fd/1 -> Divide_90fc3/2
  MathFunc_sqrt_1e51e/1 -> Subtract_64004/2
  Divide_4edae/1 -> Subtract_80558/2
  Constant_-1_0b0e9/1 -> Product_4ec73/1
  Constant_R_a_4440e/1 -> Product_4ec73/2
  Subtract_80558/1 -> Add_1c519/1
  State_psi_q_SG_D_3_ccb6a/1 -> Add_1c519/2
  Subtract_b606c/1 -> Product_ebc31/2
  Constant_R_a_73b8c/1 -> Product_0dc43/1
  Add_1c519/1 -> Product_0dc43/2
  State_psi_d_SG_D_3_1ea12/1 -> Product_1da3d/1
  State_w_SG_D_3_51c21/1 -> Product_1da3d/2
  Product_dbc38/1 -> Product_caa41/1
  Constant_f0_917b8/1 -> Product_caa41/2
  Product_ebc31/1 -> Divide_5922a/1
  Constant_x_ddd_ffb43/1 -> Divide_5922a/2
  Product_0e311/1 -> Divide_c5c1c/1
  Product_02773/1 -> Divide_c5c1c/2
  Product_0dc43/1 -> Divide_e4200/1
  Constant_x_qdd_0f11d/1 -> Divide_e4200/2
  Product_1da3d/1 -> Divide_f072a/1
  Product_caa41/1 -> Divide_f072a/2
  Divide_5922a/1 -> Add_82ac4/1
  Divide_c5c1c/1 -> Add_82ac4/2
  Divide_e4200/1 -> Add_23edd/1
  Constant_-1_848ed/1 -> Product_bad1d/1
  State_E_fd_SG_D_3_d8376/1 -> Product_bad1d/2
  Constant_2.0_3bce7/1 -> Power_52663/2
  Add_23edd/1 -> Power_95bca/1
  Product_bad1d/1 -> Product_f4862/1
  Constant_K_A_1927f/1 -> Product_f4862/2
  Constant_K_s_ba817/1 -> Product_0c01c/1
  State_Px_3_SG_D_3_c1107/1 -> Product_0c01c/2
  Power_52663/1 -> Add_0c513/1
  Power_95bca/1 -> Add_0c513/2
  Product_f4862/1 -> Product_46906/1
  Constant_K_F_256a3/1 -> Product_46906/2
  Product_0c01c/1 -> Add_8dd9b/1
  Constant_V_ref_5b646/1 -> Add_8dd9b/2
  Product_46906/1 -> Divide_dd6c3/1
  Constant_T_F_e85a5/1 -> Divide_dd6c3/2
  Add_a1229/1 -> Subtract_aca90/1
  State_R_f_SG_D_3_bcbbe/1 -> Product_0d130/2
  Divide_dd6c3/1 -> Add_e9d61/1
  Product_0d130/1 -> Add_e9d61/2
  Constant_K_A_d69a5/1 -> Product_9d02e/1
  Subtract_64004/1 -> Product_9d02e/2
  Add_e9d61/1 -> Add_a1229/1
  Product_9d02e/1 -> Add_a1229/2
  State_V_f_SG_D_3_0ee7b/1 -> Subtract_aca90/2
  Subtract_aca90/1 -> Divide_8e5da/1
  Constant_T_A_70479/1 -> Divide_8e5da/2
  Divide_8e5da/1 -> Blockout_d_V_f_SG_D_3_1ea6f/1

== system IEEE14_case/SG_D_3/d_psi_1d_SG_D_3_block ==
  note: d_psi_1d_SG_D_3 in case14gfl
      | $-\frac{\psi _{\mathrm{1d},\mathrm{SG},D,3}-\psi _{\mathrm{fd},\mathrm{SG},D,3}+\frac{\left(x_{\mathrm{dd}}-x_{l}\right)\,\left(\frac{\psi _{\mathrm{1d},\mathrm{SG},D,3}\,\left(x_{\mathrm{dd}}-x_{\mathrm{ddd}}\right)}{x_{\mathrm{dd}}-x_{l}}-\psi _{d,\mathrm{SG},D,3}+\frac{\psi _{\mathrm{fd},\mathrm{SG},D,3}\,\left(x_{\mathrm{ddd}}-x_{l}\right)}{x_{\mathrm{dd}}-x_{l}}\right)}{x_{\mathrm{ddd}}}}{T_{\mathrm{ddd}}}$
      | Automatically generated on 2025-10-09 21:32:00 .
  State_psi_1d_SG_D_3_7e8a3 : Inport
  State_psi_fd_SG_D_3_a754d : Inport  Port=2
  State_psi_1d_SG_D_3_1b7c5 : Inport  Port=3
  State_psi_d_SG_D_3_3e6ac : Inport  Port=4
  State_psi_fd_SG_D_3_e270b : Inport  Port=5
  Add_043fd : Sum
  Add_143ae : Sum
  Add_aa394 : Sum
  Constant_-1_40fda : Constant  Value=-1
  Constant_-1_ab52b : Constant  Value=-1
  Constant_T_ddd_26b07 : Constant  Value=T_ddd
  Constant_x_dd_15b27 : Constant  Value=x_dd
  Constant_x_dd_ae433 : Constant  Value=x_dd
  Constant_x_dd_d235b : Constant  Value=x_dd
  Constant_x_dd_e3d60 : Constant  Value=x_dd
  Constant_x_ddd_0b1ec : Constant  Value=x_ddd
  Constant_x_ddd_477f6 : Constant  Value=x_ddd
  Constant_x_ddd_554b1 : Constant  Value=x_ddd
  Constant_x_l_1c217 : Constant  Value=x_l
  Constant_x_l_885f2 : Constant  Value=x_l
  Constant_x_l_922af : Constant  Value=x_l
  Constant_x_l_a0eb6 : Constant  Value=x_l
  Divide_0ed84 : Product  Inputs=*/
  Divide_1d1c1 : Product  Inputs=*/
  Divide_93571 : Product  Inputs=*/
  Divide_e4ace : Product  Inputs=*/
  Product_0baa8 : Product
  Product_41967 : Product
  Product_99fd8 : Product
  Product_e97fa : Product
  Product_f1be4 : Product
  Subtract_1ba91 : Sum  Inputs=+-
  Subtract_4ef29 : Sum  Inputs=+-
  Subtract_812fd : Sum  Inputs=+-
  Subtract_a0362 : Sum  Inputs=+-
  Subtract_af01a : Sum  Inputs=+-
  Subtract_ee071 : Sum  Inputs=+-
  Blockout_d_psi_1d_SG_D_3_db4c0 : Outport
  wires:
  Divide_93571/1 -> Add_143ae/1
  Subtract_a0362/1 -> Product_f1be4/2
  Constant_-1_40fda/1 -> Product_99fd8/1
  Constant_x_dd_e3d60/1 -> Subtract_af01a/1
  State_psi_1d_SG_D_3_1b7c5/1 -> Product_99fd8/2
  Product_99fd8/1 -> Product_f1be4/1
  Constant_x_dd_15b27/1 -> Subtract_a0362/1
  Constant_x_ddd_477f6/1 -> Subtract_a0362/2
  Constant_x_l_a0eb6/1 -> Subtract_af01a/2
  Constant_x_ddd_0b1ec/1 -> Subtract_1ba91/1
  Divide_1d1c1/1 -> Blockout_d_psi_1d_SG_D_3_db4c0/1
  Constant_x_l_922af/1 -> Subtract_1ba91/2
  Product_f1be4/1 -> Divide_93571/1
  Subtract_af01a/1 -> Divide_93571/2
  State_psi_fd_SG_D_3_e270b/1 -> Product_41967/1
  Subtract_1ba91/1 -> Product_41967/2
  Constant_x_dd_d235b/1 -> Subtract_ee071/1
  Constant_x_l_1c217/1 -> Subtract_ee071/2
  State_psi_d_SG_D_3_3e6ac/1 -> Add_143ae/2
  Product_41967/1 -> Divide_0ed84/1
  Subtract_ee071/1 -> Divide_0ed84/2
  Constant_x_dd_ae433/1 -> Subtract_812fd/1
  Constant_x_l_885f2/1 -> Subtract_812fd/2
  Add_143ae/1 -> Subtract_4ef29/1
  Divide_0ed84/1 -> Subtract_4ef29/2
  Constant_-1_ab52b/1 -> Product_e97fa/1
  State_psi_1d_SG_D_3_7e8a3/1 -> Product_e97fa/2
  State_psi_fd_SG_D_3_a754d/1 -> Add_043fd/2
  Subtract_812fd/1 -> Product_0baa8/1
  Subtract_4ef29/1 -> Product_0baa8/2
  Product_e97fa/1 -> Add_043fd/1
  Product_0baa8/1 -> Divide_e4ace/1
  Constant_x_ddd_554b1/1 -> Divide_e4ace/2
  Add_043fd/1 -> Add_aa394/1
  Divide_e4ace/1 -> Add_aa394/2
  Add_aa394/1 -> Divide_1d1c1/1
  Constant_T_ddd_26b07/1 -> Divide_1d1c1/2

== system IEEE14_case/SG_D_3/d_psi_d_SG_D_3_block ==
  note: d_psi_d_SG_D_3 in case14gfl
      | $2\,\pi \,f_{0}\,\left(v_{d,\mathrm{SG},D,3}\,\sin\left(\theta _{\mathrm{SG},D,3}\right)-v_{q,\mathrm{SG},D,3}\,\cos\left(\theta _{\mathrm{SG},D,3}\right)+\frac{R_{a}\,\left(\frac{\psi _{\mathrm{1d},\mathrm{SG},D,3}\,\left(x_{\mathrm{dd}}-x_{\mathrm{ddd}}\right)}{x_{\mathrm{dd}}-x_{l}}-\psi _{d,\mathrm{SG},D,3}+\frac{\psi _{\mathrm{fd},\mathrm{SG},D,3}\,\left(x_{\mathrm{ddd}}-x_{l}\right)}{x_{\mathrm{dd}}-x_{l}}\right)}{x_{\mathrm{ddd}}}+\frac{\psi _{q,\mathrm{SG},D,3}\,w_{\mathrm{SG},D,3}}{2\,f_{0}\,\pi }\right)$
      | Automatically generated on 2025-10-09 21:31:50 .
  State_psi_1d_SG_D_3_784cd : Inport
  State_psi_d_SG_D_3_c3430 : Inport  Port=2
  State_psi_fd_SG_D_3_dc857 : Inport  Port=3
  Input_v_d_SG_D_3_50bcc : Inport  Port=4
  State_theta_SG_D_3_e69f1 : Inport  Port=5
  Input_v_q_SG_D_3_cd8a7 : Inport  Port=6
  State_theta_SG_D_3_09dff : Inport  Port=7
  State_psi_q_SG_D_3_52034 : Inport  Port=8
  State_w_SG_D_3_cf454 : Inport  Port=9
  Add_4c2c2 : Sum
  Add_6ad4f : Sum
  Constant_-1_069bf : Constant  Value=-1
  Constant_-2.0_b8c4a : Constant  Value=-2.0
  Constant_2.0_e79e2 : Constant  Value=2.0
  Constant_R_a_01cea : Constant  Value=R_a
  Constant_f0_13893 : Constant  Value=f0
  Constant_f0_bc78f : Constant  Value=f0
  Constant_pi_bfd58 : Constant  Value=pi
  Constant_pi_d83d5 : Constant  Value=pi
  Constant_x_dd_02141 : Constant  Value=x_dd
  Constant_x_dd_042d5 : Constant  Value=x_dd
  Constant_x_dd_988cd : Constant  Value=x_dd
  Constant_x_ddd_34218 : Constant  Value=x_ddd
  Constant_x_ddd_4784c : Constant  Value=x_ddd
  Constant_x_ddd_496a0 : Constant  Value=x_ddd
  Constant_x_l_a4112 : Constant  Value=x_l
  Constant_x_l_c8261 : Constant  Value=x_l
  Constant_x_l_f3092 : Constant  Value=x_l
  Divide_032f3 : Product  Inputs=*/
  Divide_22acf : Product  Inputs=*/
  Divide_850b6 : Product  Inputs=*/
  Divide_ec587 : Product  Inputs=*/
  MathFunc_cos_210e0 : Trigonometry  Operator=cos
  MathFunc_sin_22453 : Trigonometry
  Product_06488 : Product
  Product_3b0c2 : Product
  Product_45036 : Product
  Product_5e38b : Product
  Product_74280 : Product
  Product_855a2 : Product
  Product_85939 : Product
  Product_c6cde : Product
  Product_ccc08 : Product
  Product_dcc00 : Product
  Product_e2e8c : Product
  Product_f31eb : Product
  Subtract_2cef5 : Sum  Inputs=+-
  Subtract_43199 : Sum  Inputs=+-
  Subtract_76f71 : Sum  Inputs=+-
  Subtract_84f03 : Sum  Inputs=+-
  Subtract_982cc : Sum  Inputs=+-
  Subtract_c310f : Sum  Inputs=+-
  Subtract_e8495 : Sum  Inputs=+-
  Blockout_d_psi_d_SG_D_3_9ba56 : Outport
  wires:
  Constant_-1_069bf/1 -> Product_45036/1
  Constant_2.0_e79e2/1 -> Product_5e38b/1
  Constant_x_dd_02141/1 -> Subtract_2cef5/1
  State_psi_1d_SG_D_3_784cd/1 -> Product_45036/2
  Constant_x_dd_042d5/1 -> Subtract_84f03/1
  Constant_pi_bfd58/1 -> Product_5e38b/2
  Constant_x_ddd_34218/1 -> Subtract_2cef5/2
  Product_45036/1 -> Product_85939/1
  Product_5e38b/1 -> Product_ccc08/1
  Subtract_2cef5/1 -> Product_85939/2
  Constant_-2.0_b8c4a/1 -> Product_dcc00/1
  Constant_x_l_f3092/1 -> Subtract_84f03/2
  Constant_x_ddd_496a0/1 -> Subtract_e8495/1
  Constant_pi_d83d5/1 -> Product_dcc00/2
  Constant_x_l_c8261/1 -> Subtract_e8495/2
  Product_855a2/1 -> Divide_22acf/1
  Product_85939/1 -> Divide_032f3/1
  Subtract_84f03/1 -> Divide_032f3/2
  State_psi_fd_SG_D_3_dc857/1 -> Product_74280/1
  Subtract_e8495/1 -> Product_74280/2
  Constant_x_dd_988cd/1 -> Subtract_c310f/1
  Constant_x_l_a4112/1 -> Subtract_c310f/2
  Divide_22acf/1 -> Subtract_982cc/2
  Divide_032f3/1 -> Add_6ad4f/1
  Subtract_43199/1 -> Product_c6cde/2
  State_psi_d_SG_D_3_c3430/1 -> Add_6ad4f/2
  Product_74280/1 -> Divide_ec587/1
  Subtract_c310f/1 -> Divide_ec587/2
  Add_6ad4f/1 -> Subtract_43199/1
  Divide_ec587/1 -> Subtract_43199/2
  Product_e2e8c/1 -> Add_4c2c2/2
  Constant_R_a_01cea/1 -> Product_c6cde/1
  Product_06488/1 -> Product_f31eb/1
  State_theta_SG_D_3_e69f1/1 -> MathFunc_sin_22453/1
  Product_c6cde/1 -> Divide_850b6/1
  Constant_x_ddd_4784c/1 -> Divide_850b6/2
  Input_v_d_SG_D_3_50bcc/1 -> Product_3b0c2/1
  State_w_SG_D_3_cf454/1 -> Product_855a2/2
  MathFunc_sin_22453/1 -> Product_3b0c2/2
  State_theta_SG_D_3_09dff/1 -> MathFunc_cos_210e0/1
  MathFunc_cos_210e0/1 -> Product_e2e8c/2
  Divide_850b6/1 -> Subtract_76f71/1
  Product_3b0c2/1 -> Subtract_76f71/2
  Input_v_q_SG_D_3_cd8a7/1 -> Product_e2e8c/1
  State_psi_q_SG_D_3_52034/1 -> Product_855a2/1
  Constant_f0_13893/1 -> Product_ccc08/2
  Subtract_76f71/1 -> Add_4c2c2/1
  Product_ccc08/1 -> Divide_22acf/2
  Product_dcc00/1 -> Product_06488/1
  Constant_f0_bc78f/1 -> Product_06488/2
  Add_4c2c2/1 -> Subtract_982cc/1
  Subtract_982cc/1 -> Product_f31eb/2
  Product_f31eb/1 -> Blockout_d_psi_d_SG_D_3_9ba56/1
